simulink model "Dec_10_updated_33_bus_system_2MW_DG"  (R2023a)
settings: Solver=FixedStepAuto  StartTime=0.0  StopTime=0.3  RelTol=1e-3  EnableMultiTasking=on
undefined symbols (not defined in the file or in its folder): D1, Delta, DiscIntNeverNeededParam, Ts, Ts_Power
libraries: spsSeriesRLCBranchLib x42, spsThreePhaseVIMeasurementLib x35, spsThreePhaseSeriesRLCBranchLib x33, spsLoadFlowBusLib x33, spsThreePhaseParallelRLCLoadLib x31, simulink x8, spsMeanLib x5, spsFirstOrderFilterLib x4, spsStairGeneratorLib x3, spsBoostConverterLib x2, spsPowerPositiveSequenceLib x2, spsabctodq0Lib x2
(part 3 of 3)

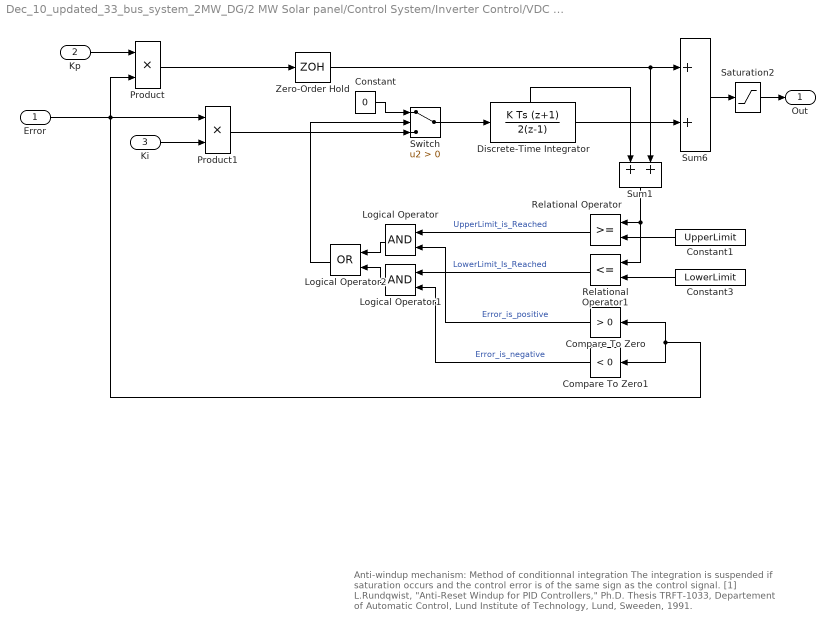
== system Dec_10_updated_33_bus_system_2MW_DG/2 MW Solar panel/Control System/Inverter Control/VDC Regulator/PI regulator with anti-windup D ==
  note: Anti-windup mechanism: Method of conditionnal integration
      |
      | The integration is suspended if saturation occurs and the
      | control error is of the same sign as the control signal.
      |
      | [1] L.Rundqwist, "Anti-Reset Windup for PID Controllers," Ph.D. Thesis TRFT-1033,
      | Departement of Automatic Control, Lund Institute of Technology, Lund, Sweeden, 1991.
  Error : Inport  SampleTime=Ts
  Kp : Inport  Port=2  SampleTime=Ts
  Ki : Inport  Port=3  SampleTime=Ts
  Compare To Zero : simulink/Logic and Bit Operations/Compare To Zero  relop=>  OutDataTypeStr=uint8  ZeroCross=off
  Compare To Zero1 : simulink/Logic and Bit Operations/Compare To Zero  relop=<  OutDataTypeStr=uint8  ZeroCross=off
  Constant : Constant  Value=0
  Constant1 : Constant  Value=UpperLimit
  Constant3 : Constant  Value=LowerLimit
  Discrete-Time Integrator : DiscreteIntegrator  IntegratorMethod=Integration: Trapezoidal  InitialCondition=Init  SampleTime=Ts  LimitOutput=on  UpperSaturationLimit=UpperLimit  LowerSaturationLimit=LowerLimit  ShowStatePort=on  ICPrevOutput=DiscIntNeverNeededParam  ICPrevScaledInput=DiscIntNeverNeededParam
  Logical Operator : Logic  AllPortsSameDT=off  OutDataTypeStr=boolean
  Logical Operator1 : Logic  AllPortsSameDT=off  OutDataTypeStr=boolean
  Logical Operator2 : Logic  Operator=OR  AllPortsSameDT=off  OutDataTypeStr=boolean
  Product : Product
  Product1 : Product
  Relational Operator : RelationalOperator  OutDataTypeStr=boolean  InputSameDT=off
  Relational Operator1 : RelationalOperator  Operator=<=  OutDataTypeStr=boolean  InputSameDT=off
  Saturation2 : Saturate  UpperLimit=UpperLimit  LowerLimit=LowerLimit  SampleTime=Ts
  Sum1 : Sum  InputSameDT=on  SaturateOnIntegerOverflow=on  SampleTime=Ts  OutDataTypeStr=Inherit: Same as first input
  Sum6 : Sum  InputSameDT=on  SaturateOnIntegerOverflow=on  SampleTime=Ts  OutDataTypeStr=Inherit: Same as first input
  Switch : Switch  Criteria=u2 > Threshold  SaturateOnIntegerOverflow=off  InputSameDT=off
  Zero-Order Hold : ZeroOrderHold  SampleTime=Ts
  Out : Outport  SampleTime=Ts  InitialOutput=0  VectorParamsAs1DForOutWhenUnconnected=off
  wires:
  Ki/1 -> Product1/2
  Kp/1 -> Product/1
  Product1/1 -> Switch/3
  Switch/1 -> Discrete-Time Integrator/1
  Saturation2/1 -> Out/1
  Discrete-Time Integrator/1 -> Sum6/2
  Product/1 -> Zero-Order Hold/1
  Sum6/1 -> Saturation2/1
  Error/1 -> Product1/1, Product/2, Compare To Zero/1, Compare To Zero1/1
  Compare To Zero1/1 -> Logical Operator1/2  "Error_is_negative"
  Logical Operator1/1 -> Logical Operator2/2
  Logical Operator/1 -> Logical Operator2/1
  Compare To Zero/1 -> Logical Operator/2  "Error_is_positive"
  Constant3/1 -> Relational Operator1/2
  Constant1/1 -> Relational Operator/2
  Relational Operator1/1 -> Logical Operator1/1  "LowerLimit_Is_Reached"
  Relational Operator/1 -> Logical Operator/1  "UpperLimit_is_Reached"
  Logical Operator2/1 -> Switch/2
  Sum1/1 -> Relational Operator/1, Relational Operator1/1
  Discrete-Time Integrator/State -> Sum1/1
  Zero-Order Hold/1 -> Sum6/1, Sum1/2
  Constant/1 -> Switch/1

== matlab function Dec_10_updated_33_bus_system_2MW_DG/2 MW Solar panel/Control System/MPPT Controller 2/MPPT Control 1  ==
  settings: updateMethod=DISCRETE  sampleTime=Ts
  data: V input =V; I input; D output; Dmax parameter; Dmin parameter; deltaD parameter; Dinit parameter
function D  = PandO(V, I, Dmax, Dmin, deltaD, Dinit)

% MPPT controller based on the Perturb & Observe algorithm.

% D output = Duty cycle of the boost converter (value between 0 and 1)
% V input = PV array terminal voltage (V)
% I input = PV array current (A)
% D = 1 - Vinput/Voutput (increasing D decrease Vin)

persistent Vold Pold Dold;
%
if isempty(Vold)
    Vold=0;
    Pold=0;
    Dold=Dinit;
end
P= V*I;
dV= V - Vold;
dP= P - Pold;
%
% if dP ~= 0
    if dP < 0
        if dV < 0
            D = Dold - deltaD;
        else
            D = Dold + deltaD;
        end
    else
        if dV < 0
            D = Dold + deltaD;
        else
            D = Dold - deltaD;
        end    
    end
% else
%     D=Dold;
% end
%
if D >= Dmax || D<= Dmin
    D=Dold;
end
%
Dold=D;
Vold=V;
Pold=P;

== matlab function Dec_10_updated_33_bus_system_2MW_DG/2 MW Solar panel/Control System/MPPT Controller 1/MPPT Control 1  ==
  settings: updateMethod=DISCRETE  sampleTime=Ts
  data: V input =V; I input; D output; Dmax parameter; Dmin parameter; deltaD parameter; Dinit parameter
function D  = PandO(V, I, Dmax, Dmin, deltaD, Dinit)

% MPPT controller based on the Perturb & Observe algorithm.

% D output = Duty cycle of the boost converter (value between 0 and 1)
% V input = PV array terminal voltage (V)
% I input = PV array current (A)
% D = 1 - Vinput/Voutput (increasing D decrease Vin)

persistent Vold Pold Dold;
%
if isempty(Vold)
    Vold=0;
    Pold=0;
    Dold=Dinit;
end
P= V*I;
dV= V - Vold;
dP= P - Pold;
%
% if dP ~= 0
    if dP < 0
        if dV < 0
            D = Dold - deltaD;
        else
            D = Dold + deltaD;
        end
    else
        if dV < 0
            D = Dold + deltaD;
        else
            D = Dold - deltaD;
        end    
    end
% else
%     D=Dold;
% end
%
if D >= Dmax || D<= Dmin
    D=Dold;
end
%
Dold=D;
Vold=V;
Pold=P;
